simulink model "Fuzzy_3i1o"  (Simulink 7.4)
settings: Solver=FixedStepDiscrete  SolverMode=SingleTasking  StartTime=0.0  StopTime=inf  FixedStep=0.002  MaxStep=0.02  RelTol=1e-3  AbsTol=1e-6
libraries: simulink x3
CloseFcn:
  | rtwprivate ssgencode ModelCloseRequest MC_AD
settings Model: Creator=fwornle  LastModifiedBy=fw  SimulationMode=external
settings ConfigSet: Description=rtmc9s12target_R2009b
settings DataIOCC: LimitDataPoints=off  SaveOutput=off  SaveTime=off  SignalLoggingName=sigsOut
settings OptimizationCC: BlockReduction=off  BooleanDataType=off  InitFltsAndDblsToZero=on  OptimizeModelRefInitCode=on  LifeSpan=1
settings DebuggingCC: SaveWithParameterizedLinksMsg=none  SignalResolutionControl=TryResolveAllWithWarning  SolverPrmCheckMsg=none  MultiTaskDSMMsg=warning  MultiTaskCondExecSysMsg=none  StrictBusMsg=None
settings HardwareCC: ProdBitPerInt=16  ProdEndianess=BigEndian  ProdWordSize=16  ProdHWDeviceType=Motorola HC12
settings RTWCC: SystemTargetFile=mc9s12.tlc  GenerateMakefile=off  TemplateMakefile=mc9s12.tmf  ProcessScript=mc9s12_make_rtw_hook  IncludeERTFirstTime=on
settings CodeAppCC: IgnoreCustomStorageClasses=off
settings STFCustomTargetCC: TargetFcnLib=ansi_tfl_tmw.mat  ModelReferenceCompliant=off  IncludeMdlTerminateFcn=off  ERTCustomFileBanners=on  SupportNonInlinedSFcns=off  CPPClassGenCompliant=on  SystemTargetFile=mc9s12.tlc
settings ERTTargetCC: TargetFcnLib=ansi_tfl_tmw.mat  MultiwordLength=2048  ModelReferenceCompliant=off  ParMdlRefBuildCompliant=off  CompOptLevelCompliant=off  IncludeMdlTerminateFcn=off  CombineOutputUpdateFcns=off  ERTFirstTimeCompliant=off  SupportContinuousTime=on  ModelStepFunctionPrototypeControlCompliant=off  ExtMode=on  ExtModeMexFile=ext_serial_mc9s12_comm  ExtModeMexArgs=1,2,115200  InlinedParameterPlacement=NonHierarchical  ERTCustomFileTemplate=mc9s12_file_process.tlc  GRTInterface=on  ConvertIfToSwitch=off
settings CustomProperty: DataType=RTWOptions_EnumType_C__Users_fw__SVN_rtmc9s12-target_trunk_rtmc9s12_CW_R2009b_bin_mc9s12_1mc9s12_TargetBoard  Value=Dragon12Plus
settings EnumStrPairs: String=Dragon12

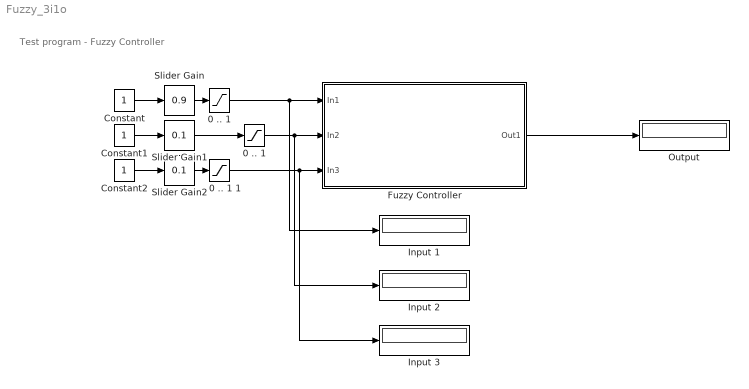
== system Fuzzy_3i1o ==
  note: Test program - Fuzzy Controller
  " 0 .. 1 " : Saturate  UpperLimit=1  LowerLimit=0
  " 0 .. 1 1" : Saturate  UpperLimit=1  LowerLimit=0
  0 .. 1 : Saturate  UpperLimit=1  LowerLimit=0
  Constant : Constant  OutDataType=sfix(16)  OutScaling=2^0
  Constant1 : Constant  OutDataType=sfix(16)  OutScaling=2^0
  Constant2 : Constant  OutDataType=sfix(16)  OutScaling=2^0
  Fuzzy Controller : Subsystem  Tag=mcTarget_fuzzy  mask{numInputs=3, MSFinput1=x1_3i1o.txt, MSFinput2=x2_3i1o.txt, MSFinput3=x3_3i1o.txt, MSFoutput=y_3i1o.txt, ruleBase=rb_3i1o.txt, sampletime=0.1}
      mask prompts: numInputs "Number of inputs"; MSFinput1 "MSFs input 1 (filename)"; MSFinput2 "MSFs input 2 (filename)"; MSFinput3 "MSFs input 3 (filename)"; MSFoutput "MSFs output (filename)"; ruleBase "Rule base (filename)"; sampletime "Sample time"
      mask init:
      | [MSFinputXstr, MSFoutputstr, ruleBasestr] = mbc_fuzzy(numInputs, MSFinput1, MSFinput2, MSFinput3, MSFoutput, ruleBase, sampletime);
      mask Help: web('fuzzy_ni1o.html');
      mask StyleString: popup(1|2|3),edit,edit,edit,edit,edit,edit
      mask Display: fprintf('%s\nMSFs output: %s\nRule base: %s', MSFinputXstr, MSFoutputstr, ruleBasestr)
  Input 1 : Display
  Input 2 : Display
  Input 3 : Display
  Output : Display
  Slider Gain : simulink/Math Operations/Slider Gain  SystemSampleTime=-1  low=0  gain=0.9  high=1
  Slider Gain1 : simulink/Math Operations/Slider Gain  SystemSampleTime=-1  low=0  gain=0.1  high=1
  Slider Gain2 : simulink/Math Operations/Slider Gain  SystemSampleTime=-1  low=0  gain=0.1  high=1
  wires:
  Constant/1 -> Slider Gain/1
  Slider Gain/1 -> 0 .. 1/1
  Constant1/1 -> Slider Gain1/1
  Fuzzy Controller/1(Out1) -> Output/1
  0 .. 1/1 -> Input 1/1, Fuzzy Controller/1(In1)
  Slider Gain1/1 -> " 0 .. 1 "/1
  " 0 .. 1 "/1 -> Input 2/1, Fuzzy Controller/2(In2)
  Constant2/1 -> Slider Gain2/1
  Slider Gain2/1 -> " 0 .. 1 1"/1
  " 0 .. 1 1"/1 -> Input 3/1, Fuzzy Controller/3(In3)

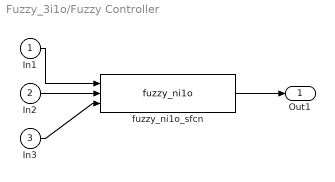
== system Fuzzy_3i1o/Fuzzy Controller ==
  In1 : Inport  OutDataType=sfix(16)  OutScaling=2^0
  In2 : Inport  Port=2  OutDataType=sfix(16)  OutScaling=2^0
  In3 : Inport  Port=3  OutDataType=sfix(16)  OutScaling=2^0
  fuzzy_ni1o_sfcn : S-Function  Tag=mcTarget_fuzzy  FunctionName=fuzzy_ni1o  Parameters=sampletime, numInputs  EnableBusSupport=off
  Out1 : Outport  OutDataType=sfix(16)  OutScaling=2^0
  wires:
  In1/1 -> fuzzy_ni1o_sfcn/1
  fuzzy_ni1o_sfcn/1 -> Out1/1
  In2/1 -> fuzzy_ni1o_sfcn/2
  In3/1 -> fuzzy_ni1o_sfcn/3
